simulink model "lista1_5a"  (R2020b)
settings: Solver=VariableStepAuto  StartTime=0.0  StopTime=10  RelTol=1e-3
settings Model: Creator=lucas  LastModifiedBy=lucas

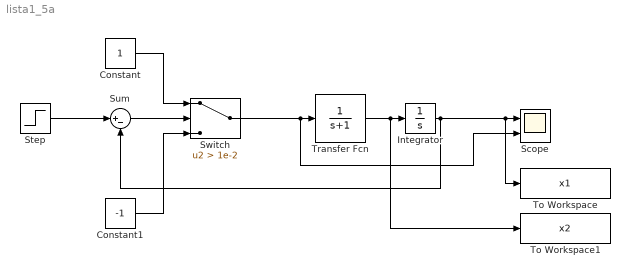
== system lista1_5a ==
  Constant : Constant
  Constant1 : Constant  Value=-1
  Integrator : Integrator
  Scope : Scope  NumInputPorts=2
  Step : Step  Time=0  SampleTime=0
  Sum : Sum  Inputs=|+-
  Switch : Switch  Criteria=u2 > Threshold  Threshold=1e-2
  To Workspace : ToWorkspace  VariableName=x1  SaveFormat=Timeseries  SampleTime=-1
  To Workspace1 : ToWorkspace  VariableName=x2  SaveFormat=Timeseries  SampleTime=-1
  Transfer Fcn : TransferFcn  Denominator=[1 1]
  wires:
  Step/1 -> Sum/1
  Sum/1 -> Switch/2
  Switch/1 -> Scope/2, Transfer Fcn/1
  Constant/1 -> Switch/1
  Constant1/1 -> Switch/3
  Transfer Fcn/1 -> To Workspace1/1, Integrator/1
  Integrator/1 -> Sum/2, To Workspace/1, Scope/1
